simulink model "AplysiaFeedingSimulation - Copy"  (R2019b)
settings: Solver=FixedStepAuto  StartTime=0.0  StopTime=40  FixedStep=0.05  RelTol=1e-3
values from neighbouring files (symbols this model uses):
  A_hinge_Init = 0.05    [AplysiaFeedingNew.m]
  A_I2_Init = 0.05    [AplysiaFeedingNew.m]
  A_I3_anterior_Init = 0.05    [AplysiaFeedingNew.m]
  A_I3_Init = 0.05    [AplysiaFeedingNew.m]
  A_I4_Init = 0.05    [AplysiaFeedingNew.m]
  B20_Init = 0    [AplysiaFeedingNew.m]
  B31B32_Init = 1    [AplysiaFeedingNew.m]
  B38_Init = 1    [AplysiaFeedingNew.m]
  B40B30_Init = 0    [AplysiaFeedingNew.m]
  B4B5_Init = 0    [AplysiaFeedingNew.m]
  B64_Init = 0    [AplysiaFeedingNew.m]
  B6B9B3_Init = 0    [AplysiaFeedingNew.m]
  B7_Init = 0    [AplysiaFeedingNew.m]
  B8_Init = 0    [AplysiaFeedingNew.m]
  c_g = 1.0    (= 1)    [AplysiaFeedingNew.m]
  c_h = 1.0    (= 1)    [AplysiaFeedingNew.m]
  CBI2_Init = 1    [AplysiaFeedingNew.m]
  CBI3_Init = 0    [AplysiaFeedingNew.m]
  CBI4_Init = 0    [AplysiaFeedingNew.m]
  fixation_type_final = 10000    [AplysiaFeedingNew.m]
  fixation_type_initial = 10000    [AplysiaFeedingNew.m]
  K_sp_g = 0.1    [AplysiaFeedingNew.m]
  K_sp_h = 2.0    (= 2)    [AplysiaFeedingNew.m]
  max_hinge = 0.2    [AplysiaFeedingNew.m]
  max_I2 = 1.5    [AplysiaFeedingNew.m]
  max_I3 = 1    [AplysiaFeedingNew.m]
  max_I3ant = 0.6    [AplysiaFeedingNew.m]
  max_I4 = 1.75    [AplysiaFeedingNew.m]
  MCC_Init = 1    [AplysiaFeedingNew.m]
  mu_k_g = 0.3    [AplysiaFeedingNew.m]
  mu_k_h = 0.3    [AplysiaFeedingNew.m]
  mu_s_g = 0.4    [AplysiaFeedingNew.m]
  mu_s_h = 0.3    [AplysiaFeedingNew.m]
  P_I3_anterior_Init = 0    [AplysiaFeedingNew.m]
  P_I4_Init = 0    [AplysiaFeedingNew.m]
  postActivityExcitation_B40B30 = 3    [AplysiaFeedingNew.m]
  seaweed_strength = 10    [AplysiaFeedingNew.m]
  sens_chemical_lips_final = 10000    [AplysiaFeedingNew.m]
  sens_chemical_lips_initial = 10000    [AplysiaFeedingNew.m]
  sens_mechanical_grasper_final = 10000    [AplysiaFeedingNew.m]
  sens_mechanical_grasper_initial = 10000    [AplysiaFeedingNew.m]
  sens_mechanical_lips_final = 10000    [AplysiaFeedingNew.m]
  sens_mechanical_lips_initial = 10000    [AplysiaFeedingNew.m]
  sensory_trigger_time = 10000    [AplysiaFeedingNew.m]
  stim_B4B5_trigger_time_end = 10000    [AplysiaFeedingNew.m]
  stim_B4B5_trigger_time_start = 10000    [AplysiaFeedingNew.m]
  stim_CBI2_trigger_time_end = 10000    [AplysiaFeedingNew.m]
  stim_CBI2_trigger_time_start = 10000    [AplysiaFeedingNew.m]
  T_hinge_Init = 0    [AplysiaFeedingNew.m]
  T_I2_Init = 0.05    [AplysiaFeedingNew.m]
  T_I3_Init = 0.05    [AplysiaFeedingNew.m]
  tau_hinge = 1.0/sqrt(2)    [AplysiaFeedingNew.m]
  tau_I2_egestion = 1.4*1/sqrt(2)    [AplysiaFeedingNew.m]
  tau_I2_ingestion = 0.5*1/sqrt(2)    [AplysiaFeedingNew.m]
  tau_I3 = 1.0/sqrt(2)    [AplysiaFeedingNew.m]
  tau_I3anterior = 2.0/sqrt(2)    [AplysiaFeedingNew.m]
  tau_I4 = 1.0/sqrt(2)    [AplysiaFeedingNew.m]
  thresh_B31_bite_off = 0.55    [AplysiaFeedingNew.m]
  thresh_B31_bite_on = 0.9    [AplysiaFeedingNew.m]
  thresh_B31_reject_off = 0.6    [AplysiaFeedingNew.m]
  thresh_B31_reject_on = 0.89    [AplysiaFeedingNew.m]
  thresh_B31_swallow_off = 0.4    [AplysiaFeedingNew.m]
  thresh_B31_swallow_on = 0.75    [AplysiaFeedingNew.m]
  thresh_B4B5_protract = 0.7    [AplysiaFeedingNew.m]
  thresh_B64_bite_protract = 0.89    [AplysiaFeedingNew.m]
  thresh_B64_reject_protract = 0.5    [AplysiaFeedingNew.m]
  thresh_B64_swallow_protract = 0.4    [AplysiaFeedingNew.m]
  thresh_B6B9B3_bite_pressure = 0.2    [AplysiaFeedingNew.m]
  thresh_B6B9B3_reject_pressure = 0.75    [AplysiaFeedingNew.m]
  thresh_B6B9B3_swallow_pressure = 0.25    [AplysiaFeedingNew.m]
  unbroken_Init = 1    [AplysiaFeedingNew.m]
  use_hypothesized_connections = 0    [AplysiaFeedingNew.m]
  x_g_Init = 0.1    [AplysiaFeedingNew.m]
  x_gh_ref = 0.4    [AplysiaFeedingNew.m]
  x_h_Init = 0    [AplysiaFeedingNew.m]
  x_h_ref = 0.0    (= 0)    [AplysiaFeedingNew.m]
(part 1 of 2)
settings Model: Creator=admin  LastModifiedBy=mecha
settings DataIOCC: ReturnWorkspaceOutputs=off

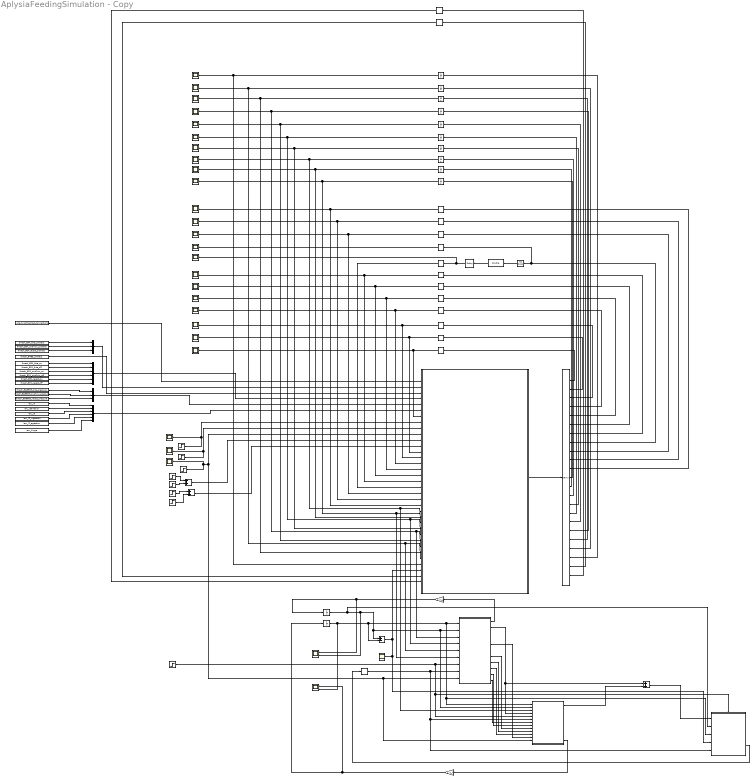
== system AplysiaFeedingSimulation - Copy ==
  Add : Sum
  Add1 : Sum  Inputs=+-
  Add2 : Sum
  Add3 : Sum
  Body Forces : Subsystem
  Cast To Double : DataTypeConversion  OutDataTypeStr=double
  Constant1 : Constant  Value=thresh_B64_bite_protract
  Constant10 : Constant  Value=thresh_B31_bite_off
  Constant11 : Constant  Value=thresh_B31_swallow_on
  Constant12 : Constant  Value=thresh_B31_swallow_off
  Constant13 : Constant  Value=thresh_B31_reject_on
  Constant14 : Constant  Value=thresh_B31_reject_off
  Constant15 : Constant  Value=thresh_B6B9B3_bite_pressure
  Constant16 : Constant  Value=thresh_B6B9B3_swallow_pressure
  Constant17 : Constant  Value=thresh_B6B9B3_reject_pressure
  Constant18 : Constant  Value=tau_I4
  Constant19 : Constant  Value=tau_I3
  Constant2 : Constant  Value=thresh_B64_swallow_protract
  Constant20 : Constant  Value=tau_I2_ingestion
  Constant21 : Constant  Value=tau_I2_egestion
  Constant22 : Constant  Value=tau_I3anterior
  Constant23 : Constant  Value=tau_hinge
  Constant3 : Constant  Value=thresh_B64_reject_protract
  Constant4 : Constant  Value=thresh_B4B5_protract
  Constant6 : Constant  Value=thresh_B31_bite_on
  Constant9 : Constant  Value=use_hypothesized_connections
  Demux1 : Demux  Outputs=23
  Enabled Subsystem : Subsystem  TreatAsAtomicUnit=on
  Gain1 : Gain  Gain=1 / c_g
  Gain2 : Gain  Gain=1 / c_h
  Grasper Forces : Subsystem
  Hit Crossing : HitCross  HitCrossingDirection=falling
  Integrator : Integrator  InitialCondition=P_I4_Init
  Integrator1 : Integrator  InitialCondition=A_I4_Init
  Integrator10 : Integrator  InitialCondition=x_h_Init
  Integrator11 : Integrator  InitialCondition=x_g_Init
  Integrator2 : Integrator  InitialCondition=T_I3_Init
  Integrator3 : Integrator  InitialCondition=A_I3_Init
  Integrator4 : Integrator  InitialCondition=T_I2_Init
  Integrator5 : Integrator  InitialCondition=A_I2_Init
  Integrator6 : Integrator  InitialCondition=P_I3_anterior_Init
  Integrator7 : Integrator  InitialCondition=A_I3_anterior_Init
  Integrator8 : Integrator  InitialCondition=T_hinge_Init
  Integrator9 : Integrator  InitialCondition=A_hinge_Init
  Memory1 : Memory  InitialCondition=B64_Init
  Memory10 : Memory  InitialCondition=B20_Init
  Memory11 : Memory  InitialCondition=B40B30_Init
  Memory12 : Memory  InitialCondition=B7_Init
  Memory13 : Memory  InitialCondition=B6B9B3_Init
  Memory14 : Memory  InitialCondition=B38_Init
  Memory15 : Memory  InitialCondition=unbroken_Init
  Memory2 : Memory  InitialCondition=B4B5_Init
  Memory3 : Memory  InitialCondition=CBI2_Init
  Memory4 : Memory  InitialCondition=MCC_Init
  Memory5 : Memory  InitialCondition=CBI3_Init
  Memory6 : Memory  InitialCondition=CBI4_Init
  Memory7 : Memory  InitialCondition=B31B32_Init
  Memory8 : Memory  InitialCondition=B40B30_Init
  Memory9 : Memory  InitialCondition=B8_Init
  Mux1 : Mux  Inputs=6
  Mux2 : Mux  Inputs=3
  Mux6 : Mux  Inputs=3
  Mux7 : Mux  Inputs=6
  Scope{,1..20,23..27} (26 alike) : Scope
  Scope21 : Scope  NumInputPorts=2
  Scope22 : Scope  NumInputPorts=2
  Step : Step  Time=sensory_trigger_time  Before=sens_mechanical_lips_initial  After=sens_mechanical_lips_final  SampleTime=0
  Step1 : Step  Time=sensory_trigger_time  Before=sens_chemical_lips_initial  After=sens_chemical_lips_final  SampleTime=0
  Step2 : Step  Time=sensory_trigger_time  Before=sens_mechanical_grasper_initial  After=sens_mechanical_grasper_final  SampleTime=0
  Step3 : Step  Time=sensory_trigger_time  Before=fixation_type_initial  After=fixation_type_final  SampleTime=0
  Step4 : Step  Time=stim_B4B5_trigger_time_start  SampleTime=0
  Step5 : Step  Time=stim_B4B5_trigger_time_end  After=-1  SampleTime=0
  Step6 : Step  Time=stim_CBI2_trigger_time_start  SampleTime=0
  Step7 : Step  Time=stim_CBI2_trigger_time_end  After=-1  SampleTime=0
  Transport Delay : TransportDelay  DelayTime=postActivityExcitation_B40B30
  neural_comp : MATLAB Function  TreatAsAtomicUnit=on
  wires:
  Grasper Forces/5(grasper_friction_state) -> Body Forces/12(grasper_friction_state)
  Integrator10/1 -> Scope22/2, Add1/2, Body Forces/1(x_h), Enabled Subsystem/3("x_h "), Grasper Forces/1(x_h)
  Step3/1 -> Enabled Subsystem/Enable, Body Forces/5(fixation_type), Grasper Forces/7(fixation_type)
  Memory15/1 -> Enabled Subsystem/5(unbroken_in), Body Forces/6(unbroken), Grasper Forces/8(unbroken)
  Grasper Forces/7(F_I3) -> Body Forces/9(F_I3)
  Grasper Forces/8(F_I4) -> Body Forces/10(F_I4)
  Grasper Forces/9(F_hinge) -> Body Forces/11(F_hinge)
  Grasper Forces/10(B2_orig) -> Body Forces/8(B2)
  Add/1 -> Enabled Subsystem/1(Force_On_Object)
  Add1/1 -> neural_comp/33(x_gh), Enabled Subsystem/4(x_gh), Scope23/1
  Enabled Subsystem/2(unbroken) -> Memory15/1
  Grasper Forces/11(A2_orig) -> Body Forces/7(A2)
  Step2/1 -> Scope10/1, Body Forces/13(sens_mechanical_grasper), Grasper Forces/9(sens_mechanical_grasper), neural_comp/10(sens_mechanical_grasper)
  neural_comp/1(y) -> Demux1/1
  Memory4/1 -> Scope7/1, neural_comp/7(MCC_In)  "MCC"
  Step1/1 -> Scope9/1, neural_comp/9(sens_chemical_lips)
  Step/1 -> Scope8/1, neural_comp/8(sens_mechanical_lips)
  Step4/1 -> Add2/1
  Step5/1 -> Add2/2
  Step6/1 -> Add3/1
  Step7/1 -> Add3/2
  Add2/1 -> neural_comp/11(stim_B4B5)
  Add3/1 -> neural_comp/12(stim_CBI2)
  Memory1/1 -> neural_comp/16(B64_In), Scope24/1  "B64"
  Memory2/1 -> Scope25/1, neural_comp/17(B4B5_In)  "B4B5"
  Constant9/1 -> neural_comp/1(use_hypothesized_connections)
  Memory3/1 -> Scope6/1, neural_comp/13(CBI2_In)  "CBI-2"
  Memory5/1 -> Scope5/1, neural_comp/14(CBI3_In)  "CBI-3"
  Memory6/1 -> Scope4/1, neural_comp/15(CBI4_In)  "CBI-4"
  Mux1/1 -> neural_comp/4(thresh_B31)
  Constant6/1 -> Mux1/1
  Constant10/1 -> Mux1/2
  Constant11/1 -> Mux1/3
  Constant12/1 -> Mux1/4
  Constant13/1 -> Mux1/5
  Constant14/1 -> Mux1/6
  Mux6/1 -> neural_comp/5(thresh_B6B9B3)
  Constant17/1 -> Mux6/3
  Constant16/1 -> Mux6/2
  Constant15/1 -> Mux6/1
  Memory13/1 -> Scope1/1, neural_comp/21(B6B9B3_In)  "B6/B9/B3"
  Integrator/1 -> Scope11/1, neural_comp/23(P_I4_In), Grasper Forces/6(P_I4)  "P_I4"
  Memory7/1 -> Scope26/1, neural_comp/20(B31B32_In)  "B31/B32"
  Integrator1/1 -> Scope12/1, neural_comp/24(A_I4_in)  "A_I4"
  Constant18/1 -> Mux7/1
  Mux7/1 -> neural_comp/6(tau)
  Memory8/1 -> neural_comp/19(B40B30_In)  "B40/B30"
  Transport Delay/1 -> Scope27/1, Memory8/1
  Hit Crossing/1 -> Cast To Double/1
  Cast To Double/1 -> Transport Delay/1
  Memory10/1 -> Scope3/1, neural_comp/18(B20_In)  "B20"
  Memory9/1 -> Scope/1, neural_comp/22(B8_In)  "B8a/b"
  Memory11/1 -> Scope2/1  "B40/B30"
  Integrator2/1 -> Scope14/1, neural_comp/27(T_I3_In), Grasper Forces/4(T_I3)  "T_I3"
  Integrator3/1 -> neural_comp/28(A_I3_In), Scope13/1  "A_I3"
  Constant19/1 -> Mux7/3
  Integrator4/1 -> Scope16/1, neural_comp/29(T_I2_In), Grasper Forces/3(T_I2)  "T_I2"
  Integrator5/1 -> neural_comp/30(A_I2_In), Scope15/1  "A_I2"
  Constant20/1 -> Mux7/4
  Constant21/1 -> Mux7/5
  Memory12/1 -> neural_comp/34(B7_In)  "B7"
  Memory14/1 -> neural_comp/35(B38_In)  "B38"
  Integrator6/1 -> Scope19/1, Body Forces/3(P_I3_anterior), neural_comp/25(P_I3_anterior_In)  "P_I3_anterior"
  Integrator7/1 -> Scope20/1, neural_comp/26(A_I3_anterior_In)  "A_I3_anterior"
  Integrator8/1 -> Scope18/1, Grasper Forces/5(T_hinge), neural_comp/31(T_hinge_In)  "T_hinge"
  Integrator9/1 -> neural_comp/32(A_hinge_In), Scope17/1  "A_hinge"
  Constant22/1 -> Mux7/2
  Constant23/1 -> Mux7/6
  Grasper Forces/2(F_f_g) -> Body Forces/4(F_f_g), Add/1
  Body Forces/1(F_f_h) -> Add/2
  Integrator11/1 -> Enabled Subsystem/2(x_g), Scope21/2, Add1/1, Body Forces/2(x_g), Grasper Forces/2(x_g)
  Grasper Forces/1(F_g) -> Gain1/1
  Gain1/1 -> Scope21/1, Integrator11/1
  Gain2/1 -> Scope22/1, Integrator10/1
  Body Forces/6(F_h) -> Gain2/1
  Constant1/1 -> Mux2/1
  Constant2/1 -> Mux2/2
  Constant3/1 -> Mux2/3
  Mux2/1 -> neural_comp/2(thresh_B64)
  Constant4/1 -> neural_comp/3(thresh_B4B5_protract)
  Demux1/1 -> Memory4/1
  Demux1/2 -> Memory3/1
  Demux1/3 -> Memory5/1
  Demux1/4 -> Memory6/1
  Demux1/5 -> Memory1/1
  Demux1/6 -> Memory2/1
  Demux1/7 -> Memory10/1
  Demux1/8 -> Memory11/1, Hit Crossing/1
  Demux1/22 -> Memory12/1
  Demux1/23 -> Memory14/1
  Demux1/9 -> Memory7/1
  Demux1/10 -> Memory13/1
  Demux1/11 -> Memory9/1
  Demux1/12 -> Integrator/1
  Demux1/13 -> Integrator1/1
  Demux1/14 -> Integrator6/1
  Demux1/15 -> Integrator7/1
  Demux1/16 -> Integrator2/1
  Demux1/17 -> Integrator3/1
  Demux1/18 -> Integrator4/1
  Demux1/19 -> Integrator5/1
  Demux1/20 -> Integrator8/1
  Demux1/21 -> Integrator9/1

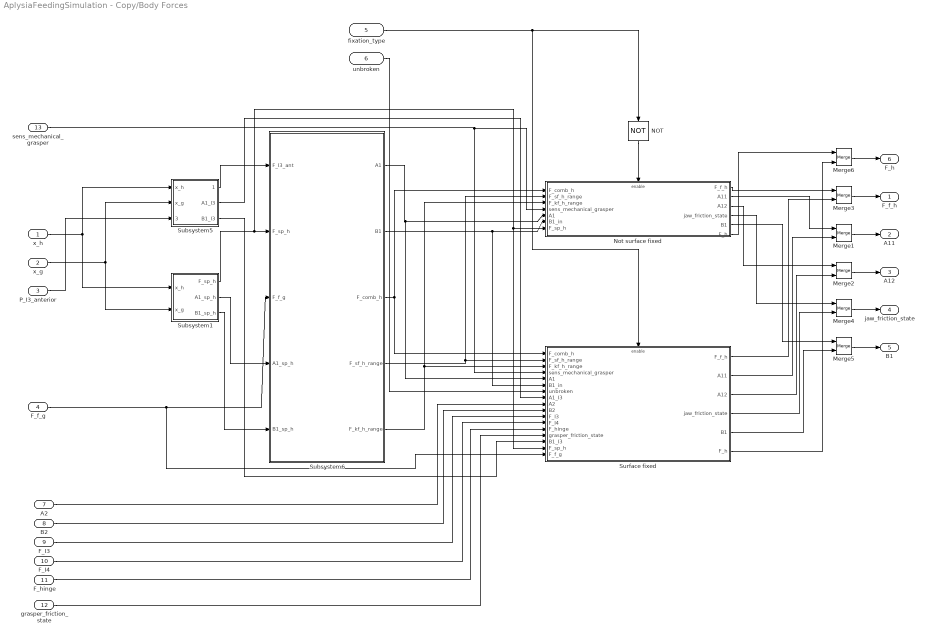
== system AplysiaFeedingSimulation - Copy/Body Forces ==
  x_h : Inport
  x_g : Inport  Port=2
  P_I3_anterior : Inport  Port=3
  F_f_g : Inport  Port=4
  fixation_type : Inport  Port=5
  unbroken : Inport  Port=6
  A2 : Inport  Port=7
  B2 : Inport  Port=8
  F_I3 : Inport  Port=9
  F_I4 : Inport  Port=10
  F_hinge : Inport  Port=11
  grasper_friction_state : Inport  Port=12
  sens_mechanical_grasper : Inport  Port=13
  Merge{1..6} (6 alike) : Merge
  NOT : Logic  Operator=NOT  IconShape=distinctive  AllPortsSameDT=off  OutDataTypeStr=boolean
  Not surface fixed : Subsystem
  Subsystem1 : Subsystem
  Subsystem5 : Subsystem
  Subsystem6 : Subsystem
  Surface fixed : Subsystem
  F_f_h : Outport
  A11 : Outport  Port=2
  A12 : Outport  Port=3
  jaw_friction_state : Outport  Port=4
  B1 : Outport  Port=5
  F_h : Outport  Port=6
  wires:
  Subsystem5/1(F_I3_ant) -> Subsystem6/1(F_I3_ant)
  Subsystem1/1(F_sp_h) -> Surface fixed/16(F_sp_h), Not surface fixed/7(F_sp_h), Subsystem6/2(F_sp_h)
  x_g/1 -> Subsystem1/2(x_g), Subsystem5/2(x_g)
  x_h/1 -> Subsystem1/1(x_h), Subsystem5/1(x_h)
  F_f_g/1 -> Surface fixed/17(F_f_g), Subsystem6/3(F_f_g)
  Subsystem6/4(F_sf_h_range) -> Not surface fixed/2(F_sf_h_range), Surface fixed/2(F_sf_h_range)
  Subsystem6/5(F_kf_h_range) -> Not surface fixed/3(F_kf_h_range), Surface fixed/3(F_kf_h_range)
  Subsystem6/1(A1) -> Surface fixed/5(A1), Not surface fixed/5(A1)
  Subsystem6/3(F_comb_h) -> Surface fixed/1(F_comb_h), Not surface fixed/1(F_comb_h)
  NOT/1 -> Not surface fixed/Enable
  fixation_type/1 -> Surface fixed/Enable, NOT/1
  Merge4/1 -> jaw_friction_state/1
  Merge1/1 -> A11/1
  Merge2/1 -> A12/1
  Merge5/1 -> B1/1
  Merge3/1 -> F_f_h/1
  Surface fixed/5(B1) -> Merge5/2
  Not surface fixed/5(B1) -> Merge5/1
  Surface fixed/4(jaw_friction_state) -> Merge4/2
  Not surface fixed/4(jaw_friction_state) -> Merge4/1
  Surface fixed/3(A12) -> Merge2/2
  Not surface fixed/3(A12) -> Merge2/1
  Surface fixed/2(A11) -> Merge1/2
  Not surface fixed/2(A11) -> Merge1/1
  Surface fixed/1(F_f_h) -> Merge3/2
  Not surface fixed/1(F_f_h) -> Merge3/1
  unbroken/1 -> Surface fixed/7(unbroken)
  Subsystem5/2(A1_I3) -> Surface fixed/8(A1_I3)
  Subsystem5/3(B1_I3) -> Surface fixed/15(B1_I3)
  Subsystem1/2(A1_sp_h) -> Subsystem6/4(A1_sp_h)
  Subsystem1/3(B1_sp_h) -> Subsystem6/5(B1_sp_h)
  A2/1 -> Surface fixed/9(A2)
  B2/1 -> Surface fixed/10(B2)
  grasper_friction_state/1 -> Surface fixed/14(grasper_friction_state)
  Subsystem6/2(B1) -> Surface fixed/6(B1_in), Not surface fixed/6(B1_in)
  P_I3_anterior/1 -> Subsystem5/3(P_I3_anterior)
  F_hinge/1 -> Surface fixed/13(F_hinge)
  F_I3/1 -> Surface fixed/11(F_I3)
  F_I4/1 -> Surface fixed/12(F_I4)
  sens_mechanical_grasper/1 -> Surface fixed/4(sens_mechanical_grasper), Not surface fixed/4(sens_mechanical_grasper)
  Merge6/1 -> F_h/1
  Not surface fixed/6(F_h) -> Merge6/1
  Surface fixed/6(F_h) -> Merge6/2

== system AplysiaFeedingSimulation - Copy/Enabled Subsystem ==
  Force_On_Object : Inport
  x_g : Inport  Port=2
  "x_h " : Inport  Port=3
  x_gh : Inport  Port=4
  unbroken_in : Inport  Port=5
  Enable : EnablePort
  AND : Logic  Inputs=3  IconShape=distinctive  AllPortsSameDT=off  OutDataTypeStr=boolean
  Add : Sum  Inputs=+-
  Constant : Constant  Value=seaweed_strength
  Constant1 : Constant  Value=0.3
  Enabled Subsystem : Subsystem  TreatAsAtomicUnit=on
  Enabled Subsystem1 : Subsystem  TreatAsAtomicUnit=on
  GreaterThan : RelationalOperator  Operator=>  OutDataTypeStr=boolean  RndMeth=Simplest
  Less Than : RelationalOperator  Operator=<  OutDataTypeStr=boolean  RndMeth=Simplest
  Less Than1 : RelationalOperator  Operator=>  OutDataTypeStr=boolean  RndMeth=Simplest
  Merge : Merge
  NOT : Logic  Operator=NOT  IconShape=distinctive  AllPortsSameDT=off  OutDataTypeStr=boolean
  NOT1 : Logic  Operator=NOT  IconShape=distinctive  AllPortsSameDT=off  OutDataTypeStr=boolean
  Product : Product
  foo : Outport
  unbroken : Outport  Port=2
  wires:
  Force_On_Object/1 -> Product/1, GreaterThan/1
  Constant/1 -> GreaterThan/2
  x_g/1 -> Add/1
  "x_h "/1 -> Add/2
  x_gh/1 -> Less Than1/2, Less Than/1
  Constant1/1 -> Less Than/2
  Add/1 -> Less Than1/1
  unbroken_in/1 -> Enabled Subsystem1/2(unbroken_in), NOT/1
  Less Than1/1 -> AND/1
  Less Than/1 -> AND/2
  NOT/1 -> AND/3
  AND/1 -> Enabled Subsystem/Enable, NOT1/1
  NOT1/1 -> Enabled Subsystem1/Enable
  GreaterThan/1 -> Enabled Subsystem1/1(force_check)
  Merge/1 -> Product/2, unbroken/1
  Enabled Subsystem1/1(Out1) -> Merge/2
  Enabled Subsystem/1(Out1) -> Merge/1
  Product/1 -> foo/1

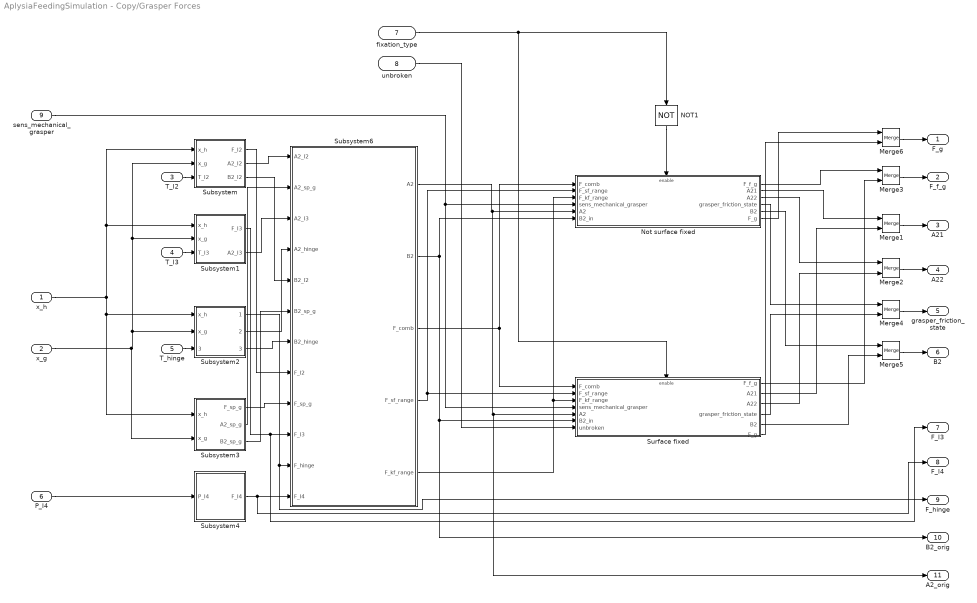
== system AplysiaFeedingSimulation - Copy/Grasper Forces ==
  x_h : Inport
  x_g : Inport  Port=2
  T_I2 : Inport  Port=3
  T_I3 : Inport  Port=4
  T_hinge : Inport  Port=5
  P_I4 : Inport  Port=6
  fixation_type : Inport  Port=7
  unbroken : Inport  Port=8
  sens_mechanical_grasper : Inport  Port=9
  Merge{1..6} (6 alike) : Merge
  NOT1 : Logic  Operator=NOT  IconShape=distinctive  AllPortsSameDT=off  OutDataTypeStr=boolean
  Not surface fixed : Subsystem
  Subsystem : Subsystem
  Subsystem1 : Subsystem
  Subsystem2 : Subsystem
  Subsystem3 : Subsystem
  Subsystem4 : Subsystem
  Subsystem6 : Subsystem
  Surface fixed : Subsystem
  F_g : Outport
  F_f_g : Outport  Port=2
  A21 : Outport  Port=3
  A22 : Outport  Port=4
  grasper_friction_state : Outport  Port=5
  B2 : Outport  Port=6
  F_I3 : Outport  Port=7
  F_I4 : Outport  Port=8
  F_hinge : Outport  Port=9
  B2_orig : Outport  Port=10
  A2_orig : Outport  Port=11
  wires:
  T_hinge/1 -> Subsystem2/3(T_hinge)
  x_h/1 -> Subsystem3/1(x_h), Subsystem2/1(x_h), Subsystem1/1(x_h), Subsystem/1(x_h)
  P_I4/1 -> Subsystem4/1(P_I4)
  x_g/1 -> Subsystem3/2(x_g), Subsystem1/2(x_g), Subsystem/2(x_g), Subsystem2/2(x_g)
  T_I3/1 -> Subsystem1/3(T_I3)
  T_I2/1 -> Subsystem/3(T_I2)
  Subsystem4/1(F_I4) -> F_I4/1, Subsystem6/12(F_I4)
  Subsystem/2(A2_I2) -> Subsystem6/1(A2_I2)
  Subsystem/1(F_I2) -> Subsystem6/8(F_I2)
  Subsystem/3(B2_I2) -> Subsystem6/5(B2_I2)
  Subsystem1/1(F_I3) -> F_I3/1, Subsystem6/10(F_I3)
  Subsystem3/1(F_sp_g) -> Subsystem6/9(F_sp_g)
  Subsystem3/2(A2_sp_g) -> Subsystem6/2(A2_sp_g)
  Subsystem3/3(B2_sp_g) -> Subsystem6/6(B2_sp_g)
  Subsystem2/1(F_hinge) -> F_hinge/1, Subsystem6/11(F_hinge)
  Subsystem2/3(B2_hinge) -> Subsystem6/7(B2_hinge)
  Subsystem2/2(A2_hinge) -> Subsystem6/4(A2_hinge)
  Subsystem1/2(A2_I3) -> Subsystem6/3(A2_I3)
  fixation_type/1 -> Surface fixed/Enable, NOT1/1
  unbroken/1 -> Surface fixed/7(unbroken)
  Subsystem6/1(A2) -> A2_orig/1, Surface fixed/5(A2), Not surface fixed/5(A2)
  Subsystem6/4(F_sf_range) -> Surface fixed/2(F_sf_range), Not surface fixed/2(F_sf_range)
  Subsystem6/5(F_kf_range) -> Not surface fixed/3(F_kf_range), Surface fixed/3(F_kf_range)
  sens_mechanical_grasper/1 -> Surface fixed/4(sens_mechanical_grasper), Not surface fixed/4(sens_mechanical_grasper)
  Merge1/1 -> A21/1
  Merge2/1 -> A22/1
  Merge4/1 -> grasper_friction_state/1
  Not surface fixed/1(F_f_g) -> Merge3/1
  Surface fixed/1(F_f_g) -> Merge3/2
  Not surface fixed/2(A21) -> Merge1/1
  Surface fixed/2(A21) -> Merge1/2
  Not surface fixed/3(A22) -> Merge2/1
  Surface fixed/3(A22) -> Merge2/2
  Not surface fixed/4(grasper_friction_state) -> Merge4/1
  Surface fixed/4(grasper_friction_state) -> Merge4/2
  Not surface fixed/5(B2) -> Merge5/1
  NOT1/1 -> Not surface fixed/Enable
  Subsystem6/2(B2) -> B2_orig/1, Surface fixed/6(B2_in), Not surface fixed/6(B2_in)
  Surface fixed/5(B2) -> Merge5/2
  Merge5/1 -> B2/1
  Subsystem6/3(F_comb) -> Surface fixed/1(F_comb), Not surface fixed/1(F_comb)
  Merge3/1 -> F_f_g/1
  Merge6/1 -> F_g/1
  Surface fixed/6(F_g) -> Merge6/2
  Not surface fixed/6(F_g) -> Merge6/1

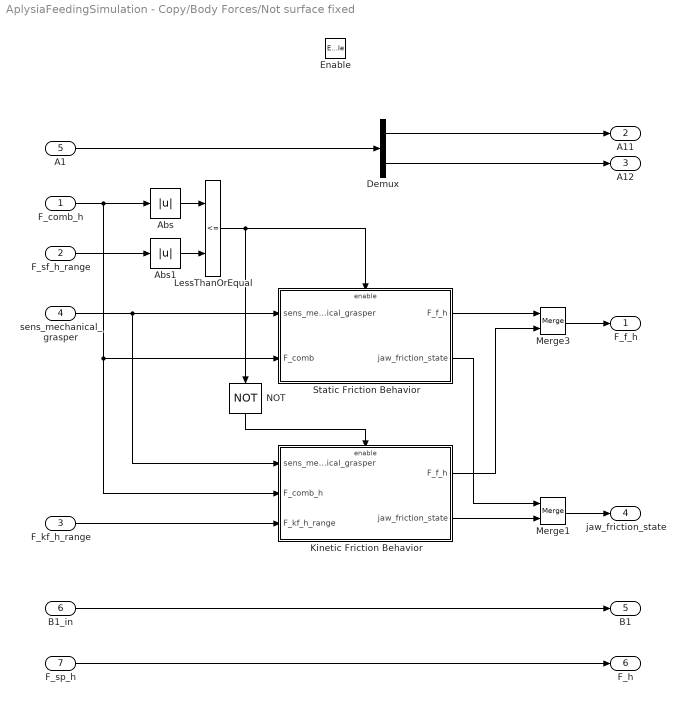
== system AplysiaFeedingSimulation - Copy/Body Forces/Not surface fixed ==
  F_comb_h : Inport
  F_sf_h_range : Inport  Port=2
  F_kf_h_range : Inport  Port=3
  sens_mechanical_grasper : Inport  Port=4
  A1 : Inport  Port=5
  B1_in : Inport  Port=6
  F_sp_h : Inport  Port=7
  Enable : EnablePort
  Abs : Abs
  Abs1 : Abs
  Demux : Demux  Outputs=2
  Kinetic Friction Behavior : Subsystem
  LessThanOrEqual : RelationalOperator  Operator=<=  OutDataTypeStr=boolean  RndMeth=Simplest
  Merge1 : Merge
  Merge3 : Merge
  NOT : Logic  Operator=NOT  IconShape=distinctive  AllPortsSameDT=off  OutDataTypeStr=boolean
  Static Friction Behavior : Subsystem
  F_f_h : Outport
  A11 : Outport  Port=2
  A12 : Outport  Port=3
  jaw_friction_state : Outport  Port=4
  B1 : Outport  Port=5
  F_h : Outport  Port=6
  wires:
  A1/1 -> Demux/1
  Demux/2 -> A12/1
  Demux/1 -> A11/1
  F_comb_h/1 -> Kinetic Friction Behavior/2(F_comb_h), Static Friction Behavior/2(F_comb), Abs/1
  F_kf_h_range/1 -> Kinetic Friction Behavior/3(F_kf_h_range)
  F_sf_h_range/1 -> Abs1/1
  Abs/1 -> LessThanOrEqual/1
  Abs1/1 -> LessThanOrEqual/2
  LessThanOrEqual/1 -> NOT/1, Static Friction Behavior/Enable
  NOT/1 -> Kinetic Friction Behavior/Enable
  sens_mechanical_grasper/1 -> Kinetic Friction Behavior/1(sens_mechanical_grasper), Static Friction Behavior/1(sens_mechanical_grasper)
  Static Friction Behavior/1(F_f_h) -> Merge3/1
  Kinetic Friction Behavior/1(F_f_h) -> Merge3/2
  Kinetic Friction Behavior/2(jaw_friction_state) -> Merge1/2
  Static Friction Behavior/2(jaw_friction_state) -> Merge1/1
  Merge3/1 -> F_f_h/1
  Merge1/1 -> jaw_friction_state/1
  B1_in/1 -> B1/1
  F_sp_h/1 -> F_h/1

== system AplysiaFeedingSimulation - Copy/Body Forces/Subsystem1 ==
  x_h : Inport
  x_g : Inport  Port=2
  Add2 : Sum
  Constant1 : Constant  Value=x_h_ref
  Constant2 : Constant  Value=[-1 0]
  Constant3 : Constant  Value=K_sp_h
  Dot Product1 : DotProduct  InputSameDT=on  OutDataTypeStr=Inherit: Inherit via internal rule
  Mux : Mux  Inputs=2
  Product1 : Product
  Product2 : Product
  Product3 : Product
  F_sp_h : Outport
  A1_sp_h : Outport  Port=2
  B1_sp_h : Outport  Port=3
  wires:
  Constant2/1 -> Product1/1, Dot Product1/1
  Dot Product1/1 -> Add2/2
  Mux/1 -> Dot Product1/2
  x_g/1 -> Mux/2
  x_h/1 -> Mux/1
  Product2/1 -> F_sp_h/1
  Add2/1 -> Product2/2
  Constant3/1 -> Product1/2, Product3/2, Product2/1
  Constant1/1 -> Product3/1, Add2/1
  Product1/1 -> A1_sp_h/1
  Product3/1 -> B1_sp_h/1

== system AplysiaFeedingSimulation - Copy/Body Forces/Subsystem5 ==
  x_h : Inport
  x_g : Inport  Port=2
  P_I3_anterior : Inport  Port=3
  Add2 : Sum
  Constant1 : Constant
  Constant2 : Constant  Value=[1 -1]
  Constant3 : Constant  Value=max_I3ant
  Dot Product : DotProduct  InputSameDT=on  OutDataTypeStr=Inherit: Inherit via internal rule
  Mux : Mux  Inputs=2
  Product1 : Product  Inputs=3
  Product2 : Product  Inputs=3
  Product3 : Product  Inputs=3
  F_I3_ant : Outport
  A1_I3 : Outport  Port=2
  B1_I3 : Outport  Port=3
  wires:
  Dot Product/1 -> Add2/2
  Mux/1 -> Dot Product/2
  x_g/1 -> Mux/2
  x_h/1 -> Mux/1
  Product2/1 -> F_I3_ant/1
  Add2/1 -> Product2/2
  Constant2/1 -> Product1/2, Dot Product/1
  Product1/1 -> A1_I3/1
  P_I3_anterior/1 -> Product3/3, Product1/3, Product2/3
  Constant1/1 -> Product3/2, Add2/1
  Constant3/1 -> Product3/1, Product1/1, Product2/1
  Product3/1 -> B1_I3/1

== system AplysiaFeedingSimulation - Copy/Body Forces/Subsystem6 ==
  F_I3_ant : Inport
  F_sp_h : Inport  Port=2
  F_f_g : Inport  Port=3
  A1_sp_h : Inport  Port=4
  B1_sp_h : Inport  Port=5
  Add : Sum
  Gain1 : Gain  Gain=1 / c_h
  Gain2 : Gain  Gain=mu_s_h
  Gain3 : Gain  Gain=mu_k_h
  Gain4 : Gain  Gain=1 / c_h
  A1 : Outport
  B1 : Outport  Port=2
  F_comb_h : Outport  Port=3
  F_sf_h_range : Outport  Port=4
  F_kf_h_range : Outport  Port=5
  wires:
  Add/1 -> F_comb_h/1
  F_I3_ant/1 -> Gain2/1, Gain3/1
  Gain2/1 -> F_sf_h_range/1
  Gain3/1 -> F_kf_h_range/1
  F_sp_h/1 -> Add/1
  F_f_g/1 -> Add/2
  Gain4/1 -> A1/1
  A1_sp_h/1 -> Gain4/1
  Gain1/1 -> B1/1
  B1_sp_h/1 -> Gain1/1

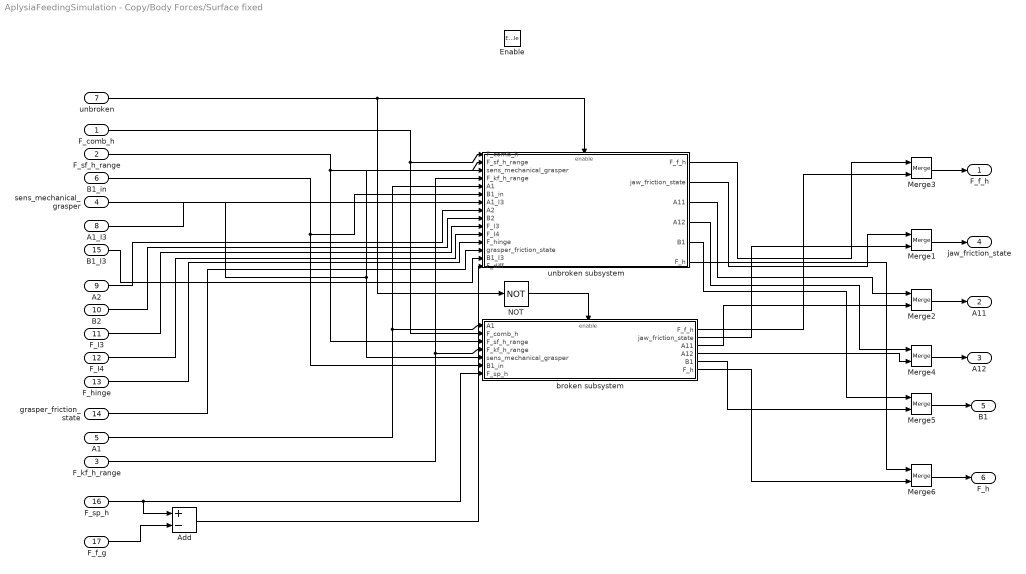
== system AplysiaFeedingSimulation - Copy/Body Forces/Surface fixed ==
  F_comb_h : Inport
  F_sf_h_range : Inport  Port=2
  F_kf_h_range : Inport  Port=3
  sens_mechanical_grasper : Inport  Port=4
  A1 : Inport  Port=5
  B1_in : Inport  Port=6
  unbroken : Inport  Port=7
  A1_I3 : Inport  Port=8
  A2 : Inport  Port=9
  B2 : Inport  Port=10
  F_I3 : Inport  Port=11
  F_I4 : Inport  Port=12
  F_hinge : Inport  Port=13
  grasper_friction_state : Inport  Port=14
  B1_I3 : Inport  Port=15
  F_sp_h : Inport  Port=16
  F_f_g : Inport  Port=17
  Enable : EnablePort
  Add : Sum  Inputs=+-
  Merge{1..6} (6 alike) : Merge
  NOT : Logic  Operator=NOT  IconShape=distinctive  AllPortsSameDT=off  OutDataTypeStr=boolean
  broken subsystem : Subsystem
  unbroken subsystem : Subsystem
  F_f_h : Outport
  A11 : Outport  Port=2
  A12 : Outport  Port=3
  jaw_friction_state : Outport  Port=4
  B1 : Outport  Port=5
  F_h : Outport  Port=6
  wires:
  unbroken/1 -> NOT/1, unbroken subsystem/Enable
  NOT/1 -> broken subsystem/Enable
  F_comb_h/1 -> broken subsystem/2(F_comb_h), unbroken subsystem/1(F_comb_h)
  F_sf_h_range/1 -> broken subsystem/3(F_sf_h_range), unbroken subsystem/2(F_sf_h_range)
  A1/1 -> unbroken subsystem/5(A1), broken subsystem/1(A1)
  B1_in/1 -> broken subsystem/6(B1_in), unbroken subsystem/6(B1_in)
  Merge3/1 -> F_f_h/1
  Merge1/1 -> jaw_friction_state/1
  broken subsystem/1(F_f_h) -> Merge3/2
  unbroken subsystem/2(jaw_friction_state) -> Merge1/1
  broken subsystem/2(jaw_friction_state) -> Merge1/2
  Merge2/1 -> A11/1
  Merge4/1 -> A12/1
  unbroken subsystem/3(A11) -> Merge2/1
  broken subsystem/3(A11) -> Merge2/2
  unbroken subsystem/4(A12) -> Merge4/1
  broken subsystem/4(A12) -> Merge4/2
  unbroken subsystem/5(B1) -> Merge5/1
  F_kf_h_range/1 -> unbroken subsystem/4(F_kf_h_range), broken subsystem/4(F_kf_h_range)
  sens_mechanical_grasper/1 -> unbroken subsystem/3(sens_mechanical_grasper), broken subsystem/5(sens_mechanical_grasper)
  Merge5/1 -> B1/1
  broken subsystem/5(B1) -> Merge5/2
  unbroken subsystem/1(F_f_h) -> Merge3/1
  A1_I3/1 -> unbroken subsystem/7(A1_I3)
  A2/1 -> unbroken subsystem/8(A2)
  B2/1 -> unbroken subsystem/9(B2)
  grasper_friction_state/1 -> unbroken subsystem/13(grasper_friction_state)
  B1_I3/1 -> unbroken subsystem/14(B1_I3)
  F_I3/1 -> unbroken subsystem/10(F_I3)
  F_hinge/1 -> unbroken subsystem/12(F_hinge)
  F_I4/1 -> unbroken subsystem/11(F_I4)
  Merge6/1 -> F_h/1
  F_sp_h/1 -> Add/1, broken subsystem/7(F_sp_h)
  broken subsystem/6(F_h) -> Merge6/2
  unbroken subsystem/6(F_h) -> Merge6/1
  F_f_g/1 -> Add/2
  Add/1 -> unbroken subsystem/15(F_diff)

== system AplysiaFeedingSimulation - Copy/Enabled Subsystem/Enabled Subsystem ==
  Enable : EnablePort
  Constant : Constant
  Out1 : Outport
  wires:
  Constant/1 -> Out1/1

== system AplysiaFeedingSimulation - Copy/Enabled Subsystem/Enabled Subsystem1 ==
  force_check : Inport
  unbroken_in : Inport  Port=2
  Enable : EnablePort
  Enabled Subsystem : Subsystem  TreatAsAtomicUnit=on
  Enabled Subsystem1 : Subsystem  TreatAsAtomicUnit=on
  Merge : Merge
  NOT : Logic  Operator=NOT  IconShape=distinctive  AllPortsSameDT=off  OutDataTypeStr=boolean
  Out1 : Outport
  wires:
  unbroken_in/1 -> Enabled Subsystem1/1(unbroken_in)
  force_check/1 -> NOT/1, Enabled Subsystem/Enable
  NOT/1 -> Enabled Subsystem1/Enable
  Merge/1 -> Out1/1
  Enabled Subsystem1/1(Out1) -> Merge/2
  Enabled Subsystem/1(Out1) -> Merge/1

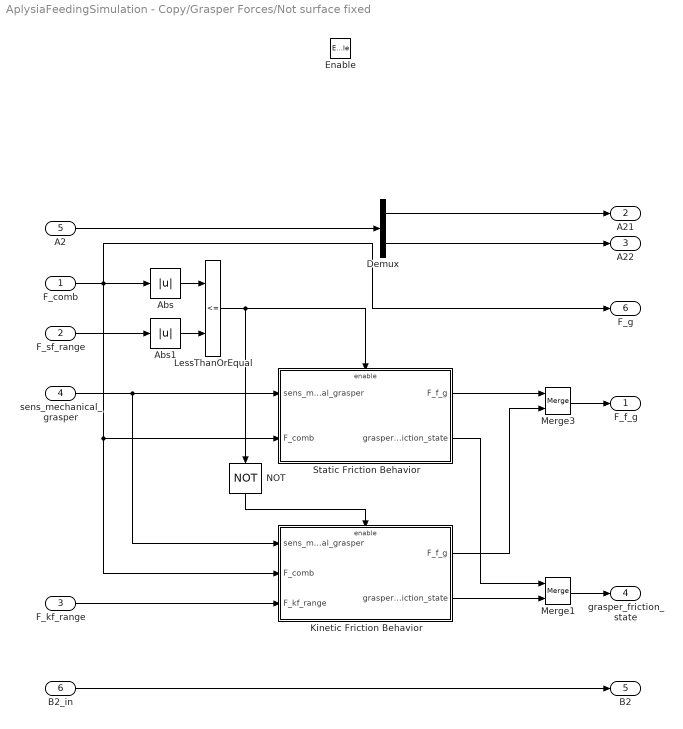
== system AplysiaFeedingSimulation - Copy/Grasper Forces/Not surface fixed ==
  F_comb : Inport
  F_sf_range : Inport  Port=2
  F_kf_range : Inport  Port=3
  sens_mechanical_grasper : Inport  Port=4
  A2 : Inport  Port=5
  B2_in : Inport  Port=6
  Enable : EnablePort
  Abs : Abs
  Abs1 : Abs
  Demux : Demux  Outputs=2
  Kinetic Friction Behavior : Subsystem
  LessThanOrEqual : RelationalOperator  Operator=<=  OutDataTypeStr=boolean  RndMeth=Simplest
  Merge1 : Merge
  Merge3 : Merge
  NOT : Logic  Operator=NOT  IconShape=distinctive  AllPortsSameDT=off  OutDataTypeStr=boolean
  Static Friction Behavior : Subsystem
  F_f_g : Outport
  A21 : Outport  Port=2
  A22 : Outport  Port=3
  grasper_friction_state : Outport  Port=4
  B2 : Outport  Port=5
  F_g : Outport  Port=6
  wires:
  A2/1 -> Demux/1
  Demux/2 -> A22/1
  Demux/1 -> A21/1
  F_comb/1 -> F_g/1, Kinetic Friction Behavior/2(F_comb), Static Friction Behavior/2(F_comb), Abs/1
  F_kf_range/1 -> Kinetic Friction Behavior/3(F_kf_range)
  F_sf_range/1 -> Abs1/1
  Abs/1 -> LessThanOrEqual/1
  Abs1/1 -> LessThanOrEqual/2
  LessThanOrEqual/1 -> NOT/1, Static Friction Behavior/Enable
  NOT/1 -> Kinetic Friction Behavior/Enable
  sens_mechanical_grasper/1 -> Kinetic Friction Behavior/1(sens_mechanical_grasper), Static Friction Behavior/1(sens_mechanical_grasper)
  Static Friction Behavior/1(F_f_g) -> Merge3/1
  Kinetic Friction Behavior/1(F_f_g) -> Merge3/2
  Kinetic Friction Behavior/2(grasper_friction_state) -> Merge1/2
  Static Friction Behavior/2(grasper_friction_state) -> Merge1/1
  Merge3/1 -> F_f_g/1
  Merge1/1 -> grasper_friction_state/1
  B2_in/1 -> B2/1

== system AplysiaFeedingSimulation - Copy/Grasper Forces/Subsystem ==
  x_h : Inport
  x_g : Inport  Port=2
  T_I2 : Inport  Port=3
  Add : Sum
  Constant : Constant  Value=max_I2
  Constant1 : Constant  Value=[1 -1]
  Constant4 : Constant
  Dot Product : DotProduct  InputSameDT=on  OutDataTypeStr=Inherit: Inherit via internal rule
  Mux : Mux  Inputs=2
  Product : Product  Inputs=3
  Product2 : Product  Inputs=3
  Product3 : Product  Inputs=3
  F_I2 : Outport
  A2_I2 : Outport  Port=2
  B2_I2 : Outport  Port=3
  wires:
  T_I2/1 -> Product3/3, Product2/3, Product/3
  Constant/1 -> Product3/1, Product2/1, Product/1
  Product/1 -> F_I2/1
  x_h/1 -> Mux/1
  x_g/1 -> Mux/2
  Constant1/1 -> Product2/2, Dot Product/1
  Mux/1 -> Dot Product/2
  Constant4/1 -> Product3/2, Add/1
  Add/1 -> Product/2
  Product2/1 -> A2_I2/1
  Product3/1 -> B2_I2/1
  Dot Product/1 -> Add/2

== system AplysiaFeedingSimulation - Copy/Grasper Forces/Subsystem1 ==
  x_h : Inport
  x_g : Inport  Port=2
  T_I3 : Inport  Port=3
  Constant1 : Constant  Value=max_I3
  Constant2 : Constant  Value=[-1 1]
  Dot Product1 : DotProduct  InputSameDT=on  OutDataTypeStr=Inherit: Inherit via internal rule
  Mux : Mux  Inputs=2
  Product : Product  Inputs=3
  Product2 : Product  Inputs=3
  F_I3 : Outport
  A2_I3 : Outport  Port=2
  wires:
  T_I3/1 -> Product2/3, Product/3
  Constant1/1 -> Product2/1, Product/1
  Product/1 -> F_I3/1
  Mux/1 -> Dot Product1/2
  Dot Product1/1 -> Product/2
  x_g/1 -> Mux/2
  x_h/1 -> Mux/1
  Constant2/1 -> Product2/2, Dot Product1/1
  Product2/1 -> A2_I3/1

== system AplysiaFeedingSimulation - Copy/Grasper Forces/Subsystem2 ==
  x_h : Inport
  x_g : Inport  Port=2
  T_hinge : Inport  Port=3
  Add2 : Sum  Inputs=-+
  Constant1 : Constant  Value=[-1 1]
  Constant2 : Constant  Value=max_hinge
  Constant3 : Constant  Value=0.5
  Dot Product1 : DotProduct  InputSameDT=on  OutDataTypeStr=Inherit: Inherit via internal rule
  GreaterThan1 : RelationalOperator  Operator=>  OutDataTypeStr=boolean  RndMeth=Simplest
  Mux : Mux  Inputs=2
  Product : Product  Inputs=4
  Product2 : Product  Inputs=4
  Product3 : Product  Inputs=4
  F_hinge : Outport
  A2_hinge : Outport  Port=2
  B2_hinge : Outport  Port=3
  wires:
  T_hinge/1 -> Product/4, Product3/4, Product2/4
  Constant2/1 -> Product/1, Product3/1, Product2/1
  Product/1 -> F_hinge/1
  Constant1/1 -> Product2/2, Dot Product1/1
  x_h/1 -> Mux/1
  x_g/1 -> Mux/2
  Mux/1 -> Dot Product1/2
  Constant3/1 -> Add2/1, Product3/2, GreaterThan1/2
  Dot Product1/1 -> GreaterThan1/1, Add2/2
  Add2/1 -> Product/2
  GreaterThan1/1 -> Product3/3, Product2/3, Product/3
  Product2/1 -> A2_hinge/1
  Product3/1 -> B2_hinge/1

== system AplysiaFeedingSimulation - Copy/Grasper Forces/Subsystem3 ==
  x_h : Inport
  x_g : Inport  Port=2
  Add : Sum
  Constant1 : Constant  Value=K_sp_g
  Constant2 : Constant  Value=[1 -1]
  Constant4 : Constant  Value=x_gh_ref
  Dot Product1 : DotProduct  InputSameDT=on  OutDataTypeStr=Inherit: Inherit via internal rule
  Mux : Mux  Inputs=2
  Product : Product
  Product2 : Product
  Product3 : Product
  F_sp_g : Outport
  A2_sp_g : Outport  Port=2
  B2_sp_g : Outport  Port=3
  wires:
  Product/1 -> F_sp_g/1
  Add/1 -> Product/1
  Constant4/1 -> Product3/1, Add/1
  Constant1/1 -> Product2/2, Product3/2, Product/2
  x_h/1 -> Mux/1
  x_g/1 -> Mux/2
  Constant2/1 -> Product2/1, Dot Product1/1
  Mux/1 -> Dot Product1/2
  Dot Product1/1 -> Add/2
  Product2/1 -> A2_sp_g/1
  Product3/1 -> B2_sp_g/1

== system AplysiaFeedingSimulation - Copy/Grasper Forces/Subsystem4 ==
  P_I4 : Inport
  Constant4 : Constant  Value=max_I4
  Product : Product
  F_I4 : Outport
  wires:
  P_I4/1 -> Product/2
  Product/1 -> F_I4/1
  Constant4/1 -> Product/1

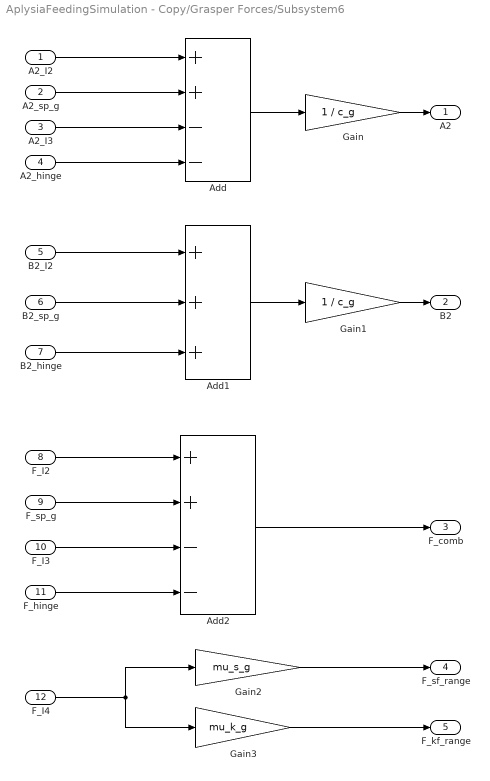
== system AplysiaFeedingSimulation - Copy/Grasper Forces/Subsystem6 ==
  A2_I2 : Inport
  A2_sp_g : Inport  Port=2
  A2_I3 : Inport  Port=3
  A2_hinge : Inport  Port=4
  B2_I2 : Inport  Port=5
  B2_sp_g : Inport  Port=6
  B2_hinge : Inport  Port=7
  F_I2 : Inport  Port=8
  F_sp_g : Inport  Port=9
  F_I3 : Inport  Port=10
  F_hinge : Inport  Port=11
  F_I4 : Inport  Port=12
  Add : Sum  Inputs=++--
  Add1 : Sum  Inputs=+++
  Add2 : Sum  Inputs=++--
  Gain : Gain  Gain=1 / c_g
  Gain1 : Gain  Gain=1 / c_g
  Gain2 : Gain  Gain=mu_s_g
  Gain3 : Gain  Gain=mu_k_g
  A2 : Outport
  B2 : Outport  Port=2
  F_comb : Outport  Port=3
  F_sf_range : Outport  Port=4
  F_kf_range : Outport  Port=5
  wires:
  A2_sp_g/1 -> Add/2
  A2_hinge/1 -> Add/4
  B2_I2/1 -> Add1/1
  B2_sp_g/1 -> Add1/2
  B2_hinge/1 -> Add1/3
  A2_I3/1 -> Add/3
  A2_I2/1 -> Add/1
  Add/1 -> Gain/1
  Add1/1 -> Gain1/1
  Gain/1 -> A2/1
  Gain1/1 -> B2/1
  F_I2/1 -> Add2/1
  F_sp_g/1 -> Add2/2
  F_I3/1 -> Add2/3
  Add2/1 -> F_comb/1
  F_I4/1 -> Gain3/1, Gain2/1
  Gain2/1 -> F_sf_range/1
  Gain3/1 -> F_kf_range/1
  F_hinge/1 -> Add2/4

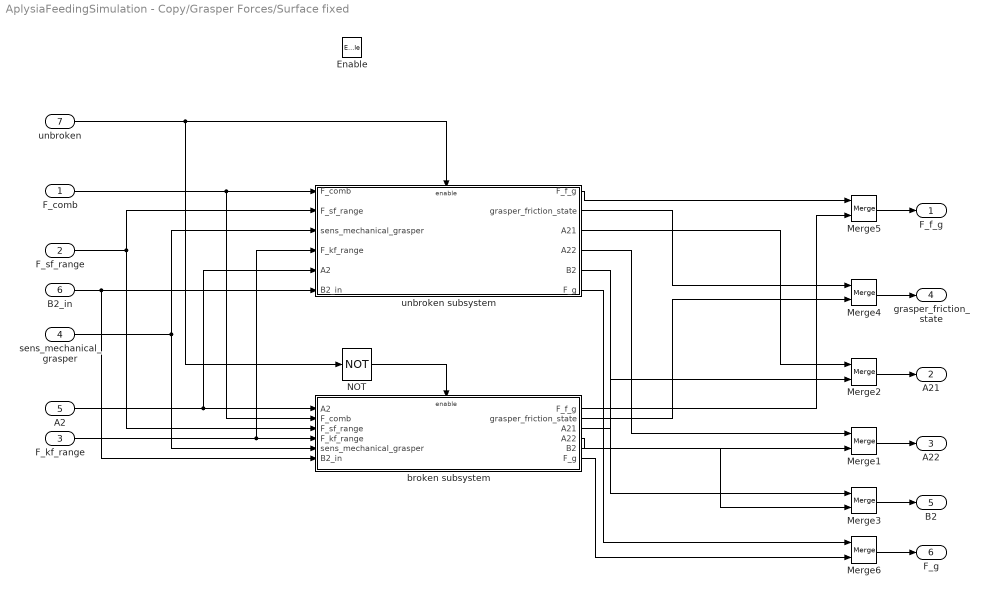
== system AplysiaFeedingSimulation - Copy/Grasper Forces/Surface fixed ==
  F_comb : Inport
  F_sf_range : Inport  Port=2
  F_kf_range : Inport  Port=3
  sens_mechanical_grasper : Inport  Port=4
  A2 : Inport  Port=5
  B2_in : Inport  Port=6
  unbroken : Inport  Port=7
  Enable : EnablePort
  Merge{1..6} (6 alike) : Merge
  NOT : Logic  Operator=NOT  IconShape=distinctive  AllPortsSameDT=off  OutDataTypeStr=boolean
  broken subsystem : Subsystem
  unbroken subsystem : Subsystem
  F_f_g : Outport
  A21 : Outport  Port=2
  A22 : Outport  Port=3
  grasper_friction_state : Outport  Port=4
  B2 : Outport  Port=5
  F_g : Outport  Port=6
  wires:
  unbroken/1 -> NOT/1, unbroken subsystem/Enable
  NOT/1 -> broken subsystem/Enable
  F_comb/1 -> broken subsystem/2(F_comb), unbroken subsystem/1(F_comb)
  F_sf_range/1 -> unbroken subsystem/2(F_sf_range), broken subsystem/3(F_sf_range)
  A2/1 -> unbroken subsystem/5(A2), broken subsystem/1(A2)
  B2_in/1 -> broken subsystem/6(B2_in), unbroken subsystem/6(B2_in)
  Merge5/1 -> F_f_g/1
  Merge4/1 -> grasper_friction_state/1
  broken subsystem/1(F_f_g) -> Merge5/2
  unbroken subsystem/2(grasper_friction_state) -> Merge4/1
  broken subsystem/2(grasper_friction_state) -> Merge4/2
  Merge2/1 -> A21/1
  Merge1/1 -> A22/1
  unbroken subsystem/3(A21) -> Merge2/1
  broken subsystem/3(A21) -> Merge2/2
  unbroken subsystem/4(A22) -> Merge1/1
  broken subsystem/4(A22) -> Merge1/2
  unbroken subsystem/5(B2) -> Merge3/1
  F_kf_range/1 -> unbroken subsystem/4(F_kf_range), broken subsystem/4(F_kf_range)
  sens_mechanical_grasper/1 -> broken subsystem/5(sens_mechanical_grasper), unbroken subsystem/3(sens_mechanical_grasper)
  Merge3/1 -> B2/1
  broken subsystem/5(B2) -> Merge3/2
  unbroken subsystem/1(F_f_g) -> Merge5/1
  Merge6/1 -> F_g/1
  broken subsystem/6(F_g) -> Merge6/2
  unbroken subsystem/6(F_g) -> Merge6/1

== system AplysiaFeedingSimulation - Copy/Body Forces/Not surface fixed/Kinetic Friction Behavior ==
  sens_mechanical_grasper : Inport
  F_comb_h : Inport  Port=2
  F_kf_h_range : Inport  Port=3
  Enable : EnablePort
  Constant : Constant  Value=0
  Gain1 : Gain  Gain=-1
  Product : Product
  Product1 : Product
  Sign : Signum
  F_f_h : Outport
  jaw_friction_state : Outport  Port=2
  wires:
  Constant/1 -> jaw_friction_state/1
  F_kf_h_range/1 -> Product/2
  Product/1 -> Product1/1
  Product1/1 -> F_f_h/1
  sens_mechanical_grasper/1 -> Product/1
  F_comb_h/1 -> Sign/1
  Sign/1 -> Gain1/1
  Gain1/1 -> Product1/2

== system AplysiaFeedingSimulation - Copy/Body Forces/Not surface fixed/Static Friction Behavior ==
  sens_mechanical_grasper : Inport
  F_comb : Inport  Port=2
  Enable : EnablePort
  Constant : Constant
  Gain : Gain  Gain=-1
  Product : Product
  F_f_h : Outport
  jaw_friction_state : Outport  Port=2
  wires:
  Constant/1 -> jaw_friction_state/1
  sens_mechanical_grasper/1 -> Gain/1
  F_comb/1 -> Product/2
  Gain/1 -> Product/1
  Product/1 -> F_f_h/1

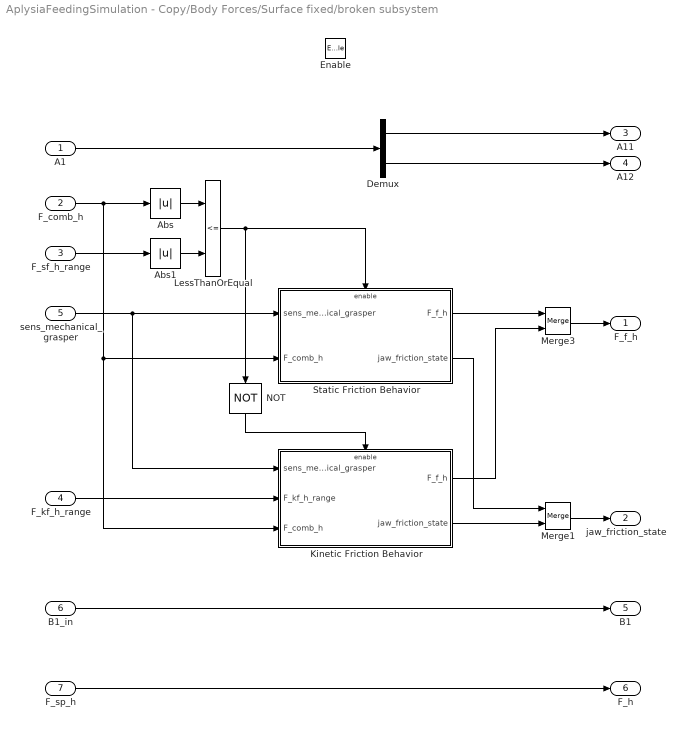
== system AplysiaFeedingSimulation - Copy/Body Forces/Surface fixed/broken subsystem ==
  A1 : Inport
  F_comb_h : Inport  Port=2
  F_sf_h_range : Inport  Port=3
  F_kf_h_range : Inport  Port=4
  sens_mechanical_grasper : Inport  Port=5
  B1_in : Inport  Port=6
  F_sp_h : Inport  Port=7
  Enable : EnablePort
  Abs : Abs
  Abs1 : Abs
  Demux : Demux  Outputs=2
  Kinetic Friction Behavior : Subsystem
  LessThanOrEqual : RelationalOperator  Operator=<=  OutDataTypeStr=boolean  RndMeth=Simplest
  Merge1 : Merge
  Merge3 : Merge
  NOT : Logic  Operator=NOT  IconShape=distinctive  AllPortsSameDT=off  OutDataTypeStr=boolean
  Static Friction Behavior : Subsystem
  F_f_h : Outport
  jaw_friction_state : Outport  Port=2
  A11 : Outport  Port=3
  A12 : Outport  Port=4
  B1 : Outport  Port=5
  F_h : Outport  Port=6
  wires:
  A1/1 -> Demux/1
  Demux/2 -> A12/1
  Demux/1 -> A11/1
  F_comb_h/1 -> Kinetic Friction Behavior/3(F_comb_h), Static Friction Behavior/2(F_comb_h), Abs/1
  F_kf_h_range/1 -> Kinetic Friction Behavior/2(F_kf_h_range)
  F_sf_h_range/1 -> Abs1/1
  Abs/1 -> LessThanOrEqual/1
  Abs1/1 -> LessThanOrEqual/2
  LessThanOrEqual/1 -> NOT/1, Static Friction Behavior/Enable
  NOT/1 -> Kinetic Friction Behavior/Enable
  sens_mechanical_grasper/1 -> Kinetic Friction Behavior/1(sens_mechanical_grasper), Static Friction Behavior/1(sens_mechanical_grasper)
  Static Friction Behavior/1(F_f_h) -> Merge3/1
  Kinetic Friction Behavior/1(F_f_h) -> Merge3/2
  Kinetic Friction Behavior/2(jaw_friction_state) -> Merge1/2
  Static Friction Behavior/2(jaw_friction_state) -> Merge1/1
  Merge3/1 -> F_f_h/1
  Merge1/1 -> jaw_friction_state/1
  B1_in/1 -> B1/1
  F_sp_h/1 -> F_h/1

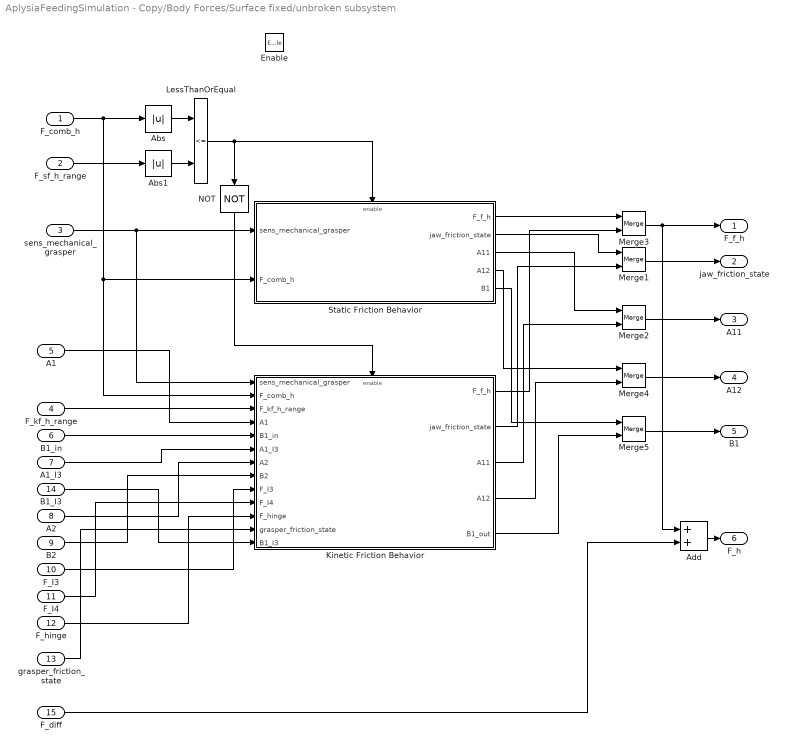
== system AplysiaFeedingSimulation - Copy/Body Forces/Surface fixed/unbroken subsystem ==
  F_comb_h : Inport
  F_sf_h_range : Inport  Port=2
  sens_mechanical_grasper : Inport  Port=3
  F_kf_h_range : Inport  Port=4
  A1 : Inport  Port=5
  B1_in : Inport  Port=6
  A1_I3 : Inport  Port=7
  A2 : Inport  Port=8
  B2 : Inport  Port=9
  F_I3 : Inport  Port=10
  F_I4 : Inport  Port=11
  F_hinge : Inport  Port=12
  grasper_friction_state : Inport  Port=13
  B1_I3 : Inport  Port=14
  F_diff : Inport  Port=15
  Enable : EnablePort
  Abs : Abs
  Abs1 : Abs
  Add : Sum
  Kinetic Friction Behavior : Subsystem
  LessThanOrEqual : RelationalOperator  Operator=<=  OutDataTypeStr=boolean  RndMeth=Simplest
  Merge{1..5} (5 alike) : Merge
  NOT : Logic  Operator=NOT  IconShape=distinctive  AllPortsSameDT=off  OutDataTypeStr=boolean
  Static Friction Behavior : Subsystem
  F_f_h : Outport
  jaw_friction_state : Outport  Port=2
  A11 : Outport  Port=3
  A12 : Outport  Port=4
  B1 : Outport  Port=5
  F_h : Outport  Port=6
  wires:
  Abs/1 -> LessThanOrEqual/1
  LessThanOrEqual/1 -> Static Friction Behavior/Enable, NOT/1
  Abs1/1 -> LessThanOrEqual/2
  Merge5/1 -> B1/1
  Merge4/1 -> A12/1
  Merge2/1 -> A11/1
  Merge1/1 -> jaw_friction_state/1
  Static Friction Behavior/1(F_f_h) -> Merge3/1
  Static Friction Behavior/2(jaw_friction_state) -> Merge1/1
  Kinetic Friction Behavior/2(jaw_friction_state) -> Merge1/2
  Static Friction Behavior/3(A11) -> Merge2/1
  Kinetic Friction Behavior/3(A11) -> Merge2/2
  Kinetic Friction Behavior/4(A12) -> Merge4/2
  Static Friction Behavior/5(B1) -> Merge5/1
  Kinetic Friction Behavior/5(B1_out) -> Merge5/2
  A1/1 -> Kinetic Friction Behavior/4(A1)
  B1_in/1 -> Kinetic Friction Behavior/5(B1_in)
  Merge3/1 -> F_f_h/1, Add/1
  F_kf_h_range/1 -> Kinetic Friction Behavior/3(F_kf_h_range)
  sens_mechanical_grasper/1 -> Static Friction Behavior/1(sens_mechanical_grasper), Kinetic Friction Behavior/1(sens_mechanical_grasper)
  Kinetic Friction Behavior/1(F_f_h) -> Merge3/2
  F_comb_h/1 -> Static Friction Behavior/2(F_comb_h), Kinetic Friction Behavior/2(F_comb_h), Abs/1
  Static Friction Behavior/4(A12) -> Merge4/1
  A1_I3/1 -> Kinetic Friction Behavior/6(A1_I3)
  A2/1 -> Kinetic Friction Behavior/7(A2)
  B2/1 -> Kinetic Friction Behavior/8(B2)
  grasper_friction_state/1 -> Kinetic Friction Behavior/12(grasper_friction_state)
  B1_I3/1 -> Kinetic Friction Behavior/13(B1_I3)
  F_I4/1 -> Kinetic Friction Behavior/10(F_I4)
  F_I3/1 -> Kinetic Friction Behavior/9(F_I3)
  F_hinge/1 -> Kinetic Friction Behavior/11(F_hinge)
  NOT/1 -> Kinetic Friction Behavior/Enable
  F_sf_h_range/1 -> Abs1/1
  Add/1 -> F_h/1
  F_diff/1 -> Add/2

== system AplysiaFeedingSimulation - Copy/Enabled Subsystem/Enabled Subsystem1/Enabled Subsystem ==
  Enable : EnablePort
  Constant : Constant  Value=0
  Out1 : Outport
  wires:
  Constant/1 -> Out1/1

== system AplysiaFeedingSimulation - Copy/Enabled Subsystem/Enabled Subsystem1/Enabled Subsystem1 ==
  unbroken_in : Inport
  Enable : EnablePort
  Out1 : Outport
  wires:
  unbroken_in/1 -> Out1/1

== system AplysiaFeedingSimulation - Copy/Grasper Forces/Not surface fixed/Kinetic Friction Behavior ==
  sens_mechanical_grasper : Inport
  F_comb : Inport  Port=2
  F_kf_range : Inport  Port=3
  Enable : EnablePort
  Abs : Abs
  Constant : Constant  Value=0
  Divide : Product  Inputs=*/
  Gain : Gain  Gain=-1
  Product : Product
  Product1 : Product
  F_f_g : Outport
  grasper_friction_state : Outport  Port=2
  wires:
  Constant/1 -> grasper_friction_state/1
  F_kf_range/1 -> Product/2
  F_comb/1 -> Abs/1, Gain/1
  Gain/1 -> Divide/1
  Abs/1 -> Divide/2
  Divide/1 -> Product1/2
  Product/1 -> Product1/1
  Product1/1 -> F_f_g/1
  sens_mechanical_grasper/1 -> Product/1

== system AplysiaFeedingSimulation - Copy/Grasper Forces/Not surface fixed/Static Friction Behavior ==
  sens_mechanical_grasper : Inport
  F_comb : Inport  Port=2
  Enable : EnablePort
  Constant : Constant
  Gain : Gain  Gain=-1
  Product : Product
  F_f_g : Outport
  grasper_friction_state : Outport  Port=2
  wires:
  Constant/1 -> grasper_friction_state/1
  sens_mechanical_grasper/1 -> Gain/1
  F_comb/1 -> Product/2
  Gain/1 -> Product/1
  Product/1 -> F_f_g/1

== system AplysiaFeedingSimulation - Copy/Grasper Forces/Surface fixed/broken subsystem ==
  A2 : Inport
  F_comb : Inport  Port=2
  F_sf_range : Inport  Port=3
  F_kf_range : Inport  Port=4
  sens_mechanical_grasper : Inport  Port=5
  B2_in : Inport  Port=6
  Enable : EnablePort
  Abs : Abs
  Abs1 : Abs
  Demux : Demux  Outputs=2
  Kinetic Friction Behavior : Subsystem
  LessThanOrEqual : RelationalOperator  Operator=<=  OutDataTypeStr=boolean  RndMeth=Simplest
  Merge1 : Merge
  Merge3 : Merge
  NOT : Logic  Operator=NOT  IconShape=distinctive  AllPortsSameDT=off  OutDataTypeStr=boolean
  Static Friction Behavior : Subsystem
  F_f_g : Outport
  grasper_friction_state : Outport  Port=2
  A21 : Outport  Port=3
  A22 : Outport  Port=4
  B2 : Outport  Port=5
  F_g : Outport  Port=6
  wires:
  A2/1 -> Demux/1
  Demux/2 -> A22/1
  Demux/1 -> A21/1
  F_comb/1 -> F_g/1, Kinetic Friction Behavior/2(F_comb), Static Friction Behavior/2(F_comb), Abs/1
  F_kf_range/1 -> Kinetic Friction Behavior/3(F_kf_range)
  F_sf_range/1 -> Abs1/1
  Abs/1 -> LessThanOrEqual/1
  Abs1/1 -> LessThanOrEqual/2
  LessThanOrEqual/1 -> NOT/1, Static Friction Behavior/Enable
  NOT/1 -> Kinetic Friction Behavior/Enable
  sens_mechanical_grasper/1 -> Kinetic Friction Behavior/1(sens_mechanical_grasper), Static Friction Behavior/1(sens_mechanical_grasper)
  Static Friction Behavior/1(F_f_g) -> Merge3/1
  Kinetic Friction Behavior/1(F_f_g) -> Merge3/2
  Kinetic Friction Behavior/2(grasper_friction_state) -> Merge1/2
  Static Friction Behavior/2(grasper_friction_state) -> Merge1/1
  Merge3/1 -> F_f_g/1
  Merge1/1 -> grasper_friction_state/1
  B2_in/1 -> B2/1

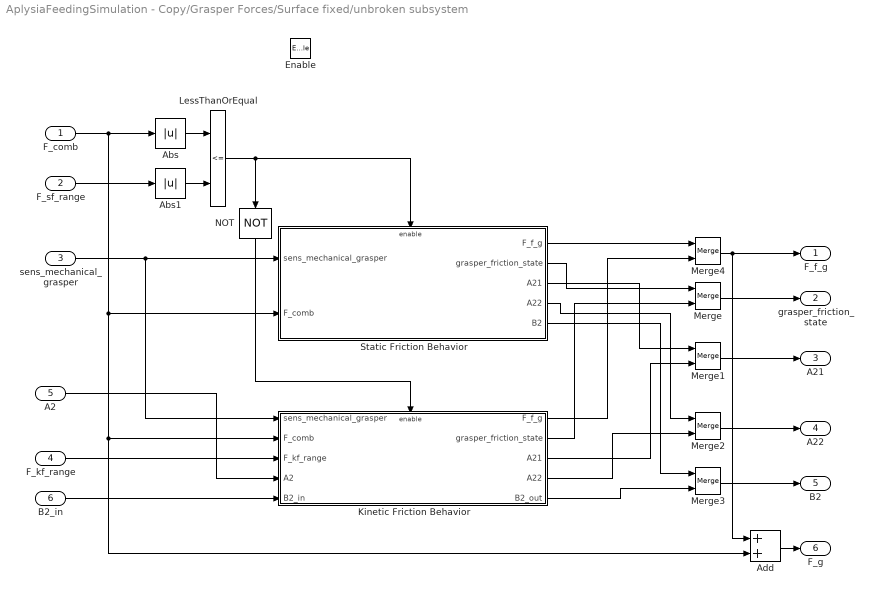
== system AplysiaFeedingSimulation - Copy/Grasper Forces/Surface fixed/unbroken subsystem ==
  F_comb : Inport
  F_sf_range : Inport  Port=2
  sens_mechanical_grasper : Inport  Port=3
  F_kf_range : Inport  Port=4
  A2 : Inport  Port=5
  B2_in : Inport  Port=6
  Enable : EnablePort
  Abs : Abs
  Abs1 : Abs
  Add : Sum
  Kinetic Friction Behavior : Subsystem
  LessThanOrEqual : RelationalOperator  Operator=<=  OutDataTypeStr=boolean  RndMeth=Simplest
  Merge{,1..4} (5 alike) : Merge
  NOT : Logic  Operator=NOT  IconShape=distinctive  AllPortsSameDT=off  OutDataTypeStr=boolean
  Static Friction Behavior : Subsystem
  F_f_g : Outport
  grasper_friction_state : Outport  Port=2
  A21 : Outport  Port=3
  A22 : Outport  Port=4
  B2 : Outport  Port=5
  F_g : Outport  Port=6
  wires:
  Abs/1 -> LessThanOrEqual/1
  LessThanOrEqual/1 -> Static Friction Behavior/Enable, NOT/1
  F_sf_range/1 -> Abs1/1
  Abs1/1 -> LessThanOrEqual/2
  NOT/1 -> Kinetic Friction Behavior/Enable
  Merge3/1 -> B2/1
  Merge2/1 -> A22/1
  Merge1/1 -> A21/1
  Merge/1 -> grasper_friction_state/1
  Static Friction Behavior/1(F_f_g) -> Merge4/1
  Static Friction Behavior/2(grasper_friction_state) -> Merge/1
  Kinetic Friction Behavior/2(grasper_friction_state) -> Merge/2
  Static Friction Behavior/3(A21) -> Merge1/1
  Kinetic Friction Behavior/3(A21) -> Merge1/2
  Kinetic Friction Behavior/4(A22) -> Merge2/2
  Static Friction Behavior/5(B2) -> Merge3/1
  Kinetic Friction Behavior/5(B2_out) -> Merge3/2
  A2/1 -> Kinetic Friction Behavior/4(A2)
  B2_in/1 -> Kinetic Friction Behavior/5(B2_in)
  Merge4/1 -> Add/1, F_f_g/1
  F_kf_range/1 -> Kinetic Friction Behavior/3(F_kf_range)
  sens_mechanical_grasper/1 -> Static Friction Behavior/1(sens_mechanical_grasper), Kinetic Friction Behavior/1(sens_mechanical_grasper)
  Kinetic Friction Behavior/1(F_f_g) -> Merge4/2
  F_comb/1 -> Static Friction Behavior/2(F_comb), Add/2, Kinetic Friction Behavior/2(F_comb), Abs/1
  Static Friction Behavior/4(A22) -> Merge2/1
  Add/1 -> F_g/1

== system AplysiaFeedingSimulation - Copy/Body Forces/Surface fixed/broken subsystem/Kinetic Friction Behavior ==
  sens_mechanical_grasper : Inport
  F_kf_h_range : Inport  Port=2
  F_comb_h : Inport  Port=3
  Enable : EnablePort
  Constant : Constant  Value=0
  Gain1 : Gain  Gain=-1
  Product : Product
  Product1 : Product
  Sign : Signum
  F_f_h : Outport
  jaw_friction_state : Outport  Port=2
  wires:
  Constant/1 -> jaw_friction_state/1
  F_kf_h_range/1 -> Product/2
  Product/1 -> Product1/1
  Product1/1 -> F_f_h/1
  sens_mechanical_grasper/1 -> Product/1
  F_comb_h/1 -> Sign/1
  Gain1/1 -> Product1/2
  Sign/1 -> Gain1/1

== system AplysiaFeedingSimulation - Copy/Body Forces/Surface fixed/broken subsystem/Static Friction Behavior ==
  sens_mechanical_grasper : Inport
  F_comb_h : Inport  Port=2
  Enable : EnablePort
  Constant : Constant
  Gain : Gain  Gain=-1
  Product : Product
  F_f_h : Outport
  jaw_friction_state : Outport  Port=2
  wires:
  Constant/1 -> jaw_friction_state/1
  sens_mechanical_grasper/1 -> Gain/1
  F_comb_h/1 -> Product/2
  Gain/1 -> Product/1
  Product/1 -> F_f_h/1
